simulink model "sim_3R_scalar"  (R2024b)
settings: Solver=FixedStepAuto  StartTime=0.0  StopTime=220  FixedStep=0.1  MaxStep=0.1  RelTol=1e-3
libraries: simulink x1
(part 2 of 2)

== matlab function sim_3R_scalar/Cluster_Controller_steepest_descent/Cluster Velocities to Cartesian Velocities ==
  data: fwdkin input; xc_err input; x1 output; zc_err input; thC_err input; a_err input; b_err input; C_err input; z1 output; th1 output; x2 output; z2 output; th2 output; x3 output; z3 output; th3 output
function [x1, z1,th1, x2,z2,th2, x3,z3, th3] = InverseJabobian(fwdkin, xc_err, zc_err, thC_err, a_err, b_err, C_err)
%% Unpacking the information from fwd_kin
p = fwdkin(1);
q = fwdkin(2);
beta = fwdkin(3);
xc = fwdkin(4);
yc = fwdkin(5);
theta_c = fwdkin(6);
yc_err = zc_err;
theta_c_err = thC_err;
p_err = a_err;
q_err = b_err;
beta_err = C_err;
%% Inverse Kinematics
  % Calculate x1, y1, and theta1 (Equations 12, 13, and 14)
r = sqrt((q + p*cos(beta))^2 + (p*sin(beta))^2);
  
x1 = xc + (1/3)*r*sin(theta_c);
y1 = yc + (1/3)*r*cos(theta_c);
%theta1 = phi1 - theta_c;
% Calculate x2, y2, and theta2 (Equations 15, 16, and 17)
x2 = xc + (1/3)*r*sin(theta_c) - p*sin(beta/2 + theta_c);
y2 = yc + (1/3)*r*cos(theta_c) - p*cos(beta/2 + theta_c);
%theta2 = phi2 - theta_c;
% Calculate x3, y3, and theta3 (Equations 18, 19, and 20)
x3 = xc + (1/3)*r*sin(theta_c) + q*sin(beta/2 - theta_c);
y3 = yc + (1/3)*r*cos(theta_c) - q*cos(beta/2 - theta_c);
%theta3 = phi3 - theta_c;
%% Now to take the partial derivates
% syms p q beta xc yc theta_c p_err q_err beta_err xc_err yc_err theta_c_err
% 
% % Define the equations
% eqs = [
%   xc + (1/3)*(sqrt((q + p*cos(beta))^2 + (p*sin(beta))^2))*sin(theta_c); % x1
%   yc + (1/3)*(sqrt((q + p*cos(beta))^2 + (p*sin(beta))^2))*cos(theta_c); % y1
%   xc + (1/3)*(sqrt((q + p*cos(beta))^2 + (p*sin(beta))^2))*sin(theta_c) - p*sin(beta/2 + theta_c); % x2
%   yc + (1/3)*(sqrt((q + p*cos(beta))^2 + (p*sin(beta))^2))*cos(theta_c) - p*cos(beta/2 + theta_c); % y2
%   xc + (1/3)*(sqrt((q + p*cos(beta))^2 + (p*sin(beta))^2))*sin(theta_c) + q*sin(beta/2 - theta_c); % x3
%   yc + (1/3)*(sqrt((q + p*cos(beta))^2 + (p*sin(beta))^2))*cos(theta_c) - q*cos(beta/2 - theta_c)  % y3
% ];
% 
% % Define the variables for differentiation
% vars = [p, q, beta, xc, yc, theta_c];
% 
% % Define the errors
% errs = [p_err, q_err, beta_err, xc_err, yc_err, theta_c_err];
% 
% % Initialize an array to store the sums (as symbolic)
% sums = sym(zeros(length(eqs), 1));
% 
% % Loop through equations and variables
% for i = 1:length(eqs)
%   for j = 1:length(vars)
%     derivative = diff(eqs(i), vars(j));
%     sums(i) = sums(i) + derivative * errs(j);
%   end
% end
% 
% % Display the results
% disp(simplify(sums(1)))
% disp(simplify(sums(2)))
% disp(simplify(sums(3)))
% disp(simplify(sums(4)))
% disp(simplify(sums(5)))
% disp(simplify(sums(6)))
%% Now to sum it all up
x1 =(3*xc_err*(p^2 + 2*cos(beta)*p*q + q^2)^(1/2) + p*p_err*sin(theta_c) + q*q_err*sin(theta_c) + p^2*theta_c_err*cos(theta_c) + q^2*theta_c_err*cos(theta_c) + p*q_err*cos(beta)*sin(theta_c) + p_err*q*cos(beta)*sin(theta_c) + 2*p*q*theta_c_err*cos(beta)*cos(theta_c) - beta_err*p*q*sin(beta)*sin(theta_c))/(3*(p^2 + 2*cos(beta)*p*q + q^2)^(1/2));
 
z1 = (3*yc_err*(p^2 + 2*cos(beta)*p*q + q^2)^(1/2) + p*p_err*cos(theta_c) + q*q_err*cos(theta_c) - p^2*theta_c_err*sin(theta_c) - q^2*theta_c_err*sin(theta_c) + p*q_err*cos(beta)*cos(theta_c) + p_err*q*cos(beta)*cos(theta_c) - beta_err*p*q*sin(beta)*cos(theta_c) - 2*p*q*theta_c_err*cos(beta)*sin(theta_c))/(3*(p^2 + 2*cos(beta)*p*q + q^2)^(1/2));
 
x2 = xc_err - p_err*(sin(beta/2 + theta_c) - (sin(theta_c)*(p + q*cos(beta)))/(3*(p^2 + 2*cos(beta)*p*q + q^2)^(1/2))) - beta_err*((p*cos(beta/2 + theta_c))/2 + (p*q*sin(beta)*sin(theta_c))/(3*(p^2 + 2*cos(beta)*p*q + q^2)^(1/2))) + theta_c_err*((cos(theta_c)*(p^2 + 2*cos(beta)*p*q + q^2)^(1/2))/3 - p*cos(beta/2 + theta_c)) + (q_err*sin(theta_c)*(q + p*cos(beta)))/(3*(p^2 + 2*cos(beta)*p*q + q^2)^(1/2));
 
z2 = yc_err - p_err*(cos(beta/2 + theta_c) - (cos(theta_c)*(p + q*cos(beta)))/(3*(p^2 + 2*cos(beta)*p*q + q^2)^(1/2))) + beta_err*((p*sin(beta/2 + theta_c))/2 - (p*q*sin(beta)*cos(theta_c))/(3*(p^2 + 2*cos(beta)*p*q + q^2)^(1/2))) - (theta_c_err*sin(theta_c)*(p^2 + 2*cos(beta)*p*q + q^2)^(1/2))/3 + p*theta_c_err*sin(beta/2 + theta_c) + (q_err*cos(theta_c)*(q + p*cos(beta)))/(3*(p^2 + 2*cos(beta)*p*q + q^2)^(1/2));
 
x3 = xc_err + q_err*(sin(beta/2 - theta_c) + (sin(theta_c)*(q + p*cos(beta)))/(3*(p^2 + 2*cos(beta)*p*q + q^2)^(1/2))) + beta_err*((q*cos(beta/2 - theta_c))/2 - (p*q*sin(beta)*sin(theta_c))/(3*(p^2 + 2*cos(beta)*p*q + q^2)^(1/2))) + (theta_c_err*cos(theta_c)*(p^2 + 2*cos(beta)*p*q + q^2)^(1/2))/3 - q*theta_c_err*cos(beta/2 - theta_c) + (p_err*sin(theta_c)*(p + q*cos(beta)))/(3*(p^2 + 2*cos(beta)*p*q + q^2)^(1/2));
 
z3 = yc_err - theta_c_err*(q*sin(beta/2 - theta_c) + (sin(theta_c)*(p^2 + 2*cos(beta)*p*q + q^2)^(1/2))/3) - q_err*(cos(beta/2 - theta_c) - (cos(theta_c)*(q + p*cos(beta)))/(3*(p^2 + 2*cos(beta)*p*q + q^2)^(1/2))) + beta_err*((q*sin(beta/2 - theta_c))/2 - (p*q*sin(beta)*cos(theta_c))/(3*(p^2 + 2*cos(beta)*p*q + q^2)^(1/2))) + (p_err*cos(theta_c)*(p + q*cos(beta)))/(3*(p^2 + 2*cos(beta)*p*q + q^2)^(1/2));
 
th1 = 0;
th2 = 0;
th3 = 0;
